simulink model "model4_linear"  (R2025b)
settings: Solver=ode23t  StartTime=0.0  StopTime=10  MaxStep=4e-5  RelTol=1e-3
undefined symbols (not defined in the file): current_con_ts, DiscIntNeverNeededParam, lin_current_con_Ki, lin_current_con_Kp, lin_dc_voltage_source, lin_gear_ratio, lin_lead, lin_motor_P_pole_pairs, lin_motor_P_rotorJ, lin_motor_P_statorLd, lin_motor_P_statorLq, lin_position_con_Kp, lin_velocity_con_Ki, lin_velocity_con_Kp, position_con_ts, velocity_con_ts
libraries: nesl_utility x11, fl_lib x9, ee_lib x7, mcbeeMathTransformLib x4, slpidlib x4, sdl_lib x1
settings Model: DataDictionary=model4_lin_data.sldd  Creator=HP-PC  LastModifiedBy=HP-PC
settings SolverCC: AutoInsertRateTranBlk=on  InsertRTBMode=Never (minimum delay)

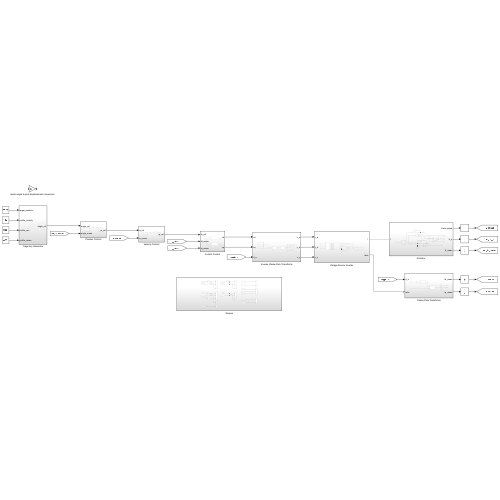
[thumbnail: Simulink's stored preview of the top-level diagram]
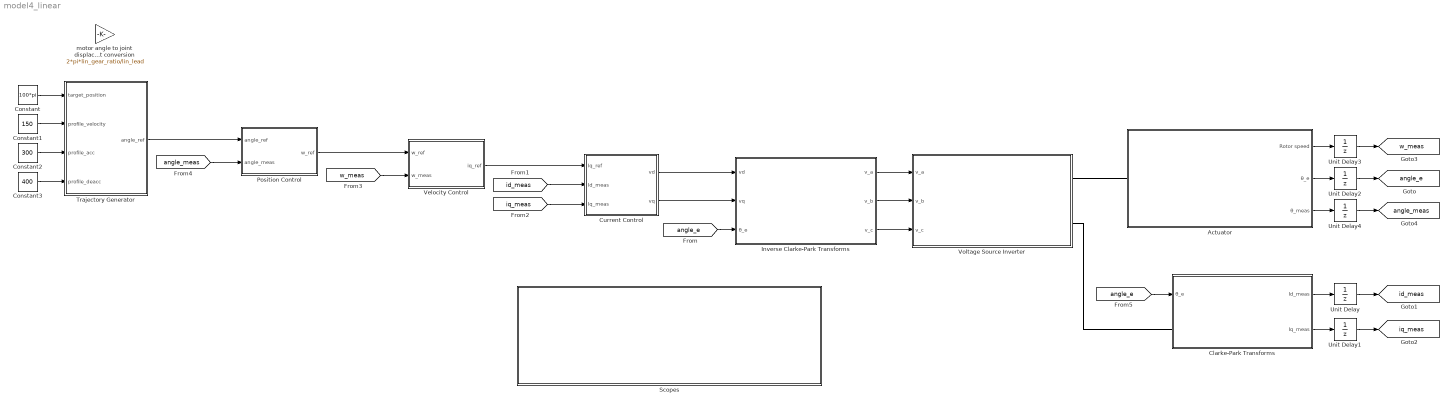
== system model4_linear ==
  Actuator : Subsystem
  Clarke-Park Transforms : Subsystem
  Constant : Constant  Value=100*pi
  Constant1 : Constant  Value=150
  Constant2 : Constant  Value=300
  Constant3 : Constant  Value=400
  Current Control : Subsystem
  Inverse Clarke-Park Transforms : Subsystem
  Position Control : Subsystem
  Scopes : Subsystem
  Trajectory Generator : Subsystem
  Unit Delay : UnitDelay  SampleTime=4e-5  HasFrameUpgradeWarning=on
  Unit Delay1 : UnitDelay  SampleTime=4e-5  HasFrameUpgradeWarning=on
  Unit Delay2 : UnitDelay  SampleTime=4e-5  HasFrameUpgradeWarning=on
  Unit Delay3 : UnitDelay  SampleTime=4e-4  HasFrameUpgradeWarning=on
  Unit Delay4 : UnitDelay  SampleTime=4e-4  HasFrameUpgradeWarning=on
  Velocity Control : Subsystem
  Voltage Source Inverter : Subsystem
  motor angle to joint displacement conversion : Gain  Gain=2*pi*lin_gear_ratio/lin_lead
  tag scope: angle_e=global, angle_meas=global, id_meas=global, iq_meas=global, w_meas=global
  wires:
  Inverse Clarke-Park Transforms/1(v_a) -> Voltage Source Inverter/1(v_a)
  Inverse Clarke-Park Transforms/2(v_b) -> Voltage Source Inverter/2(v_b)
  Inverse Clarke-Park Transforms/3(v_c) -> Voltage Source Inverter/3(v_c)
  Current Control/1(vd) -> Inverse Clarke-Park Transforms/1(vd)
  Current Control/2(vq) -> Inverse Clarke-Park Transforms/2(vq)
  Clarke-Park Transforms/1(Id_meas) -> Unit Delay/1
  Clarke-Park Transforms/2(Iq_meas) -> Unit Delay1/1
  Actuator/2(θ_e) -> Unit Delay2/1
  Unit Delay2/1 -> [angle_e]
  [angle_e] -> Inverse Clarke-Park Transforms/3(θ_e)
  Unit Delay/1 -> [id_meas]
  Unit Delay1/1 -> [iq_meas]
  [id_meas] -> Current Control/2(Id_meas)
  [iq_meas] -> Current Control/3(Iq_meas)
  Actuator/1(Rotor speed) -> Unit Delay3/1
  Unit Delay3/1 -> [w_meas]
  [w_meas] -> Velocity Control/2(w_meas)
  Position Control/1(w_ref) -> Velocity Control/1(w_ref)
  Actuator/3(θ_meas) -> Unit Delay4/1
  Unit Delay4/1 -> [angle_meas]
  [angle_meas] -> Position Control/2(angle_meas)
  Constant1/1 -> Trajectory Generator/2(profile_velocity)
  Constant2/1 -> Trajectory Generator/3(profile_acc)
  Constant3/1 -> Trajectory Generator/4(profile_deacc)
  Trajectory Generator/1(angle_ref) -> Position Control/1(angle_ref)
  Constant/1 -> Trajectory Generator/1(target_position)
  [angle_e] -> Clarke-Park Transforms/1(θ_e)
  Velocity Control/1(iq_ref) -> Current Control/1(Iq_ref)
  connections:
  Actuator/LConn1 -- Voltage Source Inverter/RConn1
  Voltage Source Inverter/RConn2 -- Clarke-Park Transforms/LConn1

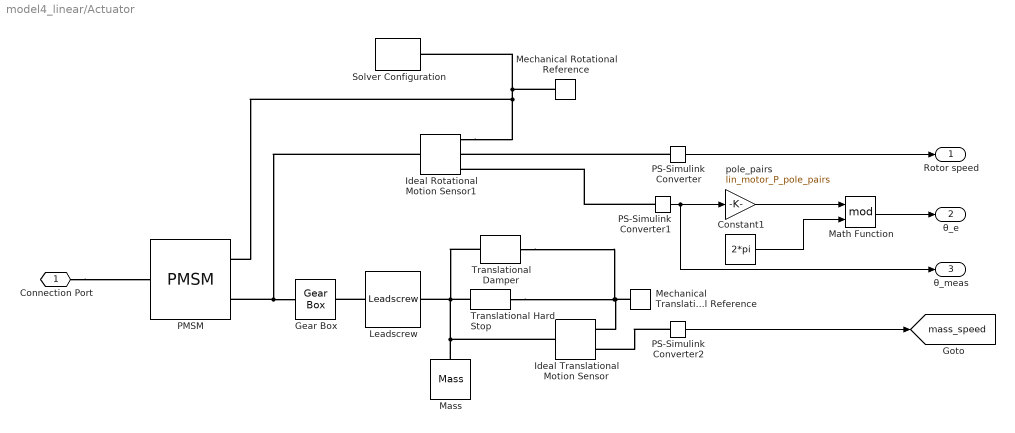
== system model4_linear/Actuator ==
  Constant1 : Constant  Value=2*pi
  Gear Box : fl_lib/Mechanical/Mechanisms/Gear Box  ratio=lin_gear_ratio  t_in_specify=off  t_in_priority=None  t_in=0 N*m  t_in_nominal_specify=off  t_in_nominal_value=1  t_in_nominal_unit=N*m  t_out_specify=off  t_out_priority=None  t_out=0 N*m  t_out_nominal_specify=off  t_out_nominal_value=1  t_out_nominal_unit=N*m
  Ideal Rotational Motion Sensor1 : fl_lib/Mechanical/Mechanical Sensors/Ideal Rotational Motion Sensor  reference=foundation.enum.MeasurementReference.difference  acceleration_port=false  velocity_port=true  position_port=true  wrap_angle=false  offset=0 rad
  Ideal Translational Motion Sensor : fl_lib/Mechanical/Mechanical Sensors/Ideal Translational Motion Sensor  reference=foundation.enum.MeasurementReference.difference  acceleration_port=false  velocity_port=true  position_port=false  offset=0 m
      settings: InternalSimscapePortConfiguration="{\"Bottom\":[],\"Left\":[{\"id\":\"R\",\"label\":\"R\",\"type\":\"foundation.mechanical.translational.translational\"}],\"Right\":[{\"id\":\"C\",\"label\":\"C\",\"type\":\"foundation.mechanical.translational.translational\"},{\"id\":\"V\",\"label\":\"V\",\"type\":\"output\"}],\"Top\":[]}"
  Leadscrew : sdl_lib/Gears/Rotational- Translational/Leadscrew  Lead=lin_lead m  helix_type=sdl.enum.handedness.right  friction_model=sdl.enum.gear_friction.constant  friction_parameterization=sdl.enum.frictionParameterization.efficiencies  lambda=15 deg  alpha=14.5 deg  fr_coeff=0.08  eff_sn=lin_screwnut_efficiency  eff_ns=lin_screwnut_efficiency  temperature_TLU=[280, 300, 320] K  efficiency_sn_TLU=[.75, .65, .6]  efficiency_ns_TLU=[.5, .45, .4]  pwr_thr=0.001 W  mu_visc=0 N*m*s/rad  thermal_mass=50 J/K  temperature_specify=off  temperature_priority=High  temperature=300 K  temperature_nominal_specify=off  temperature_nominal_value=1  temperature_nominal_unit=K
      settings: InternalSimscapePortConfiguration="{\"Bottom\":[],\"Left\":[{\"id\":\"S\",\"label\":\"S\",\"type\":\"foundation.mechanical.rotational.rotational\"}],\"Right\":[{\"id\":\"N\",\"label\":\"N\",\"type\":\"foundation.mechanical.translational.translational\"}],\"Top\":[]}"
  Mass : fl_lib/Mechanical/Translational Elements/Mass  mass=1 kg  num_ports=foundation.enum.numPorts2.one  v_specify=off  v_priority=High  v=0 m/s  v_nominal_specify=off  v_nominal_value=1  v_nominal_unit=m/s  f_specify=off  f_priority=None  f=0 N  f_nominal_specify=off  f_nominal_value=1  f_nominal_unit=N
  Math Function : Math  Operator=mod
  Mechanical Rotational Reference : fl_lib/Mechanical/Rotational Elements/Mechanical Rotational Reference
  Mechanical Translational Reference : fl_lib/Mechanical/Translational Elements/Mechanical Translational Reference
  PMSM : ee_lib/Electromechanical/Permanent Magnet/PMSM  port_option=ee.enum.threePhasePort.composite  winding_type=ee.enum.electromech.statorconfiguration.wye  machine_param=ee.enum.pmsm.parameterization.constant  nPolePairs=lin_motor_P_pole_pairs  pmflux_param=ee.enum.pmflux.torqueconstant  pm_flux_linkage=0.03 Wb  torque_constant=lin_motor_P_torqueK N*m/A  back_emf_constant=0.18 V*s/rad  stator_param=ee.enum.statorparam.LdLqL0  Ld=lin_motor_P_statorLd H  Lq=lin_motor_P_statorLq H  idVec=[-200, 0, 200] A  iqVec=[-200, 0, 200] A  LdMatrix=0.0002 * ones(3, 3) H  LqMatrix=0.0002 * ones(3, 3) H  PmMatrix=0.1 * ones(3, 3) Wb  ktMatrix=0.18 * ones(3, 3) N*m/A  keMatrix=0.18 * ones(3, 3) V*s/rad  L0=0.00016 H  Ls=0.0002 H  Lm=-0.00002 H  Ms=0.00002 H  Rs=lin_motor_P_statorR Ohm  zero_sequence=ee.enum.park.zerosequence.exclude  axes_param=ee.enum.rotorangle.daxis  loss_param=ee.enum.ironloss.none  losses_oc=[0, 0, 0] W  losses_sc=[0, 0, 0] W  f_losses=60 Hz  Isc_losses=95 A  J=lin_motor_P_rotorJ kg*m^2  lam=0 N*m*s/rad  i_d_specify=off  i_d_priority=None  i_d=0 A  i_d_nominal_specify=off  i_d_nominal_value=1  i_d_nominal_unit=A  i_q_specify=off  i_q_priority=None  i_q=0 A  i_q_nominal_specify=off  i_q_nominal_value=1  i_q_nominal_unit=A  torque_specify=off  torque_priority=None  torque=0 N*m  torque_nominal_specify=off  torque_nominal_value=1  torque_nominal_unit=N*m  angular_velocity_specify=off  angular_velocity_priority=High  angular_velocity=0 rpm  angular_velocity_nominal_specify=off  angular_velocity_nominal_value=1  angular_velocity_nominal_unit=rpm  angular_position_specify=off  angular_position_priority=High  angular_position=0 deg  angular_position_nominal_specify=off  angular_position_nominal_value=1  angular_position_nominal_unit=deg  alpha=3.93e-3 1/K  alpha_flux=-0.001 1/K  Tmeas=298.15 K  stator_thermal_mass=100 J/K  rotor_thermal_mass=200 J/K  Rm_percent_rotor=90  Rd_percent_rotor=30  temperatureA_specify=off  temperatureA_priority=High  temperatureA=25 degC  temperatureA_nominal_specify=off  temperatureA_nominal_value=1  temperatureA_nominal_unit=degC  temperatureB_specify=off  temperatureB_priority=High  temperatureB=25 degC  temperatureB_nominal_specify=off  temperatureB_nominal_value=1  temperatureB_nominal_unit=degC  temperatureC_specify=off  temperatureC_priority=High  temperatureC=25 degC  temperatureC_nominal_specify=off  temperatureC_nominal_value=1  temperatureC_nominal_unit=degC  temperatureR_specify=off  temperatureR_priority=High  temperatureR=25 degC  temperatureR_nominal_specify=off  temperatureR_nominal_value=1  temperatureR_nominal_unit=degC
      settings: InternalSimscapePortConfiguration="{\"Bottom\":[],\"Left\":[{\"id\":\"N\",\"label\":\"~\",\"type\":\"foundation.electrical.three_phase\"}],\"Right\":[{\"id\":\"R\",\"label\":\"R\",\"type\":\"foundation.mechanical.rotational.rotational\"},{\"id\":\"C\",\"label\":\"C\",\"type\":\"foundation.mechanical.rotational.rotational\"}],\"Top\":[]}"
  PS-Simulink Converter : nesl_utility/PS-Simulink Converter  PhysicalDomain=network_engine_domain  SubClassName=ps_output  LeftPortType=input  RightPortType=output  PseudoPeriodic=off  Frequencies=[]  VectorFormat=inherit  Unit=rad/s  AffineConversion=off
  PS-Simulink Converter1 : nesl_utility/PS-Simulink Converter  PhysicalDomain=network_engine_domain  SubClassName=ps_output  LeftPortType=input  RightPortType=output  PseudoPeriodic=off  Frequencies=[]  VectorFormat=inherit  Unit=rad  AffineConversion=off
  PS-Simulink Converter2 : nesl_utility/PS-Simulink Converter  PhysicalDomain=network_engine_domain  SubClassName=ps_output  LeftPortType=input  RightPortType=output  PseudoPeriodic=off  Frequencies=[]  VectorFormat=inherit  Unit=inherit  AffineConversion=off
  Solver Configuration : nesl_utility/Solver Configuration  PhysicalDomain=network_engine_domain  SubClassName=solver  LeftPortType=input  RightPortType=generic  Tones=[]  Harmonics=[]  SimulateNoise=off  Profile=off  UseLocalSampling=off  EnableSwitchedLinearOptims=on  FrequencyDomain=off  UseCCode=off  RelTol=0.001  AbsTol=0.001  MinStep=1e-09  ToWorkspace=off  RevertToSquareIcSolve=off  NumHomotopyIterations=100  PhasorMode=off  PhasorModeNumHarmonics=1  ConsistencySolver=NEWTON_XTOL_AFTER_FTOL  IndexReductionMethod=DerivativeReplacement  DoDC=off  ResidualTolerance=1e-09  ConsistencyTolSource=GLOBAL  ConsistencyAbsTol=0.001  ConsistencyRelTol=0.001  ConsistencyTolFactor=0.001  UseLocalSolver=off  LocalSolverChoice=NE_BACKWARD_EULER_ADVANCER  ResolveIndetEquations=on  FunctionEvalNumThread=1  LocalSolverSampleTime=0.001  DoFixedCost=off  MaxNonlinIter=3  MaxModeIter=2  ComputeImpulses=off  ImpulseIterations=2  LinearAlgebra=auto  LinearAlgebraNumThread=0  EquationFormulation=NE_TIME_EF  DelaysMemoryBudget=1024  AutomaticFiltering=on  FilteringTimeConstant=0.001  PartitionStorageMethod=AS_NEEDED  PartitionMemoryBudget=1024  PartitionMethod=ROBUST  MultibodyUseLocalSolver=off  MultibodyLocalSolverChoice=ODE1  MultibodyLocalSolverSampleTime=0.001
  Translational Damper : fl_lib/Mechanical/Translational Elements/Translational Damper  D=10 N*s/m  v_specify=off  v_priority=None  v=0 m/s  v_nominal_specify=off  v_nominal_value=1  v_nominal_unit=m/s  f_specify=off  f_priority=None  f=0 N  f_nominal_specify=off  f_nominal_value=1  f_nominal_unit=N
  Translational Hard Stop : fl_lib/Mechanical/Translational Elements/Translational Hard Stop  upper_bnd=0.05 m  lower_bnd=-0.05 m  model=simscape.enum.hardstop.smooth  stiff_up=1e6 N/m  stiff_low=1e6 N/m  D_up=150 N*s/m  D_low=150 N*s/m  transition=0.1 mm  coeff_rest=0.7  v_tol=0.001 m/s  f_tol=0.001 N  v_specify=off  v_priority=None  v=0 m/s  v_nominal_specify=off  v_nominal_value=1  v_nominal_unit=m/s  f_specify=off  f_priority=None  f=0 N  f_nominal_specify=off  f_nominal_value=1  f_nominal_unit=N  x_specify=off  x_priority=High  x=0 m  x_nominal_specify=off  x_nominal_value=1  x_nominal_unit=m  M_specify=off  M_priority=None  M=0
  pole_pairs : Gain  Gain=lin_motor_P_pole_pairs
  Connection Port : PMIOPort  Side=Left
  Rotor speed : Outport
  θ_e : Outport  Port=2
  θ_meas : Outport  Port=3
  tag scope: mass_speed=global
  wires:
  PS-Simulink Converter/1 -> Rotor speed/1
  pole_pairs/1 -> Math Function/1
  Constant1/1 -> Math Function/2
  PS-Simulink Converter1/1 -> θ_meas/1, pole_pairs/1
  Math Function/1 -> θ_e/1
  PS-Simulink Converter2/1 -> [mass_speed]
  connections:
  Mechanical Rotational Reference/LConn1 -- Ideal Rotational Motion Sensor1/RConn1 -- PMSM/RConn2 -- Solver Configuration/RConn1
  PS-Simulink Converter/LConn1 -- Ideal Rotational Motion Sensor1/RConn2
  Connection Port/RConn1 -- PMSM/LConn1
  Ideal Rotational Motion Sensor1/LConn1 -- Gear Box/LConn1 -- PMSM/RConn1
  PS-Simulink Converter1/LConn1 -- Ideal Rotational Motion Sensor1/RConn3
  Leadscrew/LConn1 -- Gear Box/RConn1
  Translational Damper/LConn1 -- Ideal Translational Motion Sensor/LConn1 -- Mass/LConn1 -- Leadscrew/RConn1 -- Translational Hard Stop/LConn1
  Mechanical Translational Reference/LConn1 -- Translational Hard Stop/RConn1 -- Translational Damper/RConn1 -- Ideal Translational Motion Sensor/RConn1
  PS-Simulink Converter2/LConn1 -- Ideal Translational Motion Sensor/RConn2

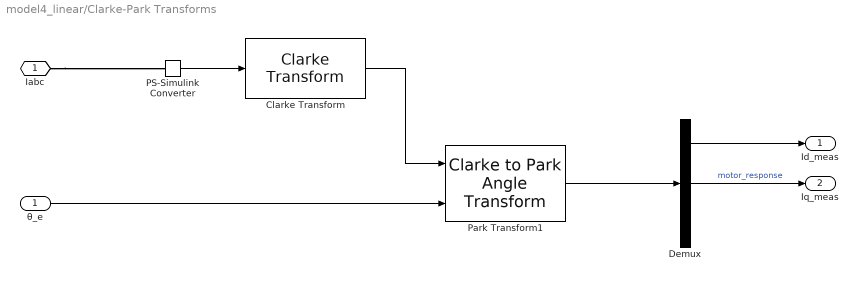
== system model4_linear/Clarke-Park Transforms ==
  θ_e : Inport
  Clarke Transform : mcbeeMathTransformLib/Clarke Transform  VariantControl=Variant2  PowerInvariant=off  UseWithEmbedded=on  PhaseInput=Three inputs
      settings: LibrarySourceBlock=mcblib/Controls/Math Transforms/Clarke Transform
  Demux : Demux  Outputs=3
  PS-Simulink Converter : nesl_utility/PS-Simulink Converter  PhysicalDomain=network_engine_domain  SubClassName=ps_output  LeftPortType=input  RightPortType=output  PseudoPeriodic=off  Frequencies=[]  VectorFormat=inherit  Unit=inherit  AffineConversion=off
  Park Transform1 : mcbeeMathTransformLib/Clarke to Park Angle Transform  AxisAlignment=D-axis  UseWithEmbedded=on  PhaseInput=Three inputs  ThetaInput=Electrical position  AngleInput=Radians  N_points=1024
      settings: LibrarySourceBlock=mcblib/Controls/Math Transforms/Park Transform
  Iabc : PMIOPort  Side=Left
  Id_meas : Outport
  Iq_meas : Outport  Port=2
  wires:
  PS-Simulink Converter/1 -> Clarke Transform/1
  Clarke Transform/1 -> Park Transform1/1
  Park Transform1/1 -> Demux/1
  Demux/1 -> Id_meas/1
  Demux/2 -> Iq_meas/1  "motor_response"
  θ_e/1 -> Park Transform1/2
  connections:
  Iabc/RConn1 -- PS-Simulink Converter/LConn1

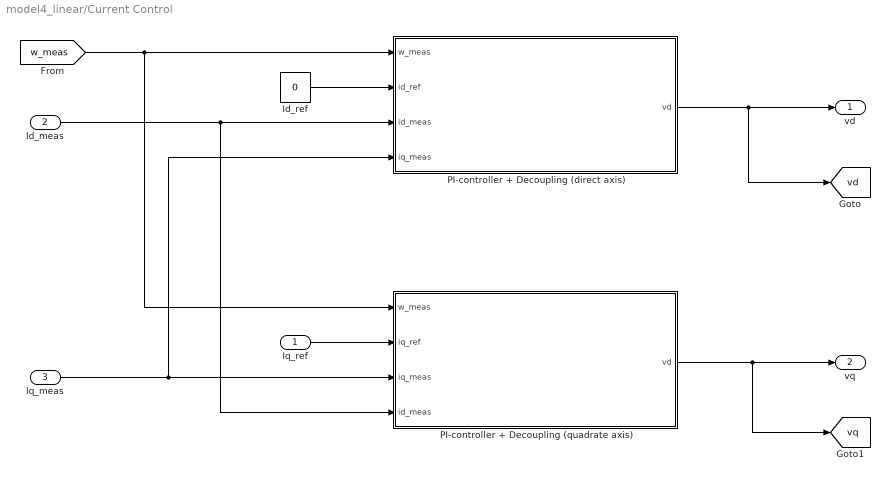
== system model4_linear/Current Control ==
  Iq_ref : Inport
  Id_meas : Inport  Port=2
  Iq_meas : Inport  Port=3
  Id_ref : Constant  Value=0
  PI-controller + Decoupling (direct axis) : Subsystem
  PI-controller + Decoupling (quadrate axis) : Subsystem
  vd : Outport
  vq : Outport  Port=2
  tag scope: vd=global, vq=global
  wires:
  [w_meas] -> PI-controller + Decoupling (quadrate axis)/1(w_meas), PI-controller + Decoupling (direct axis)/1(w_meas)
  Id_ref/1 -> PI-controller + Decoupling (direct axis)/2(id_ref)
  Id_meas/1 -> PI-controller + Decoupling (quadrate axis)/4(id_meas), PI-controller + Decoupling (direct axis)/3(id_meas)
  PI-controller + Decoupling (quadrate axis)/1(vd) -> [vq], vq/1
  PI-controller + Decoupling (direct axis)/1(vd) -> [vd], vd/1
  Iq_ref/1 -> PI-controller + Decoupling (quadrate axis)/2(iq_ref)
  Iq_meas/1 -> PI-controller + Decoupling (direct axis)/4(iq_meas), PI-controller + Decoupling (quadrate axis)/3(iq_meas)

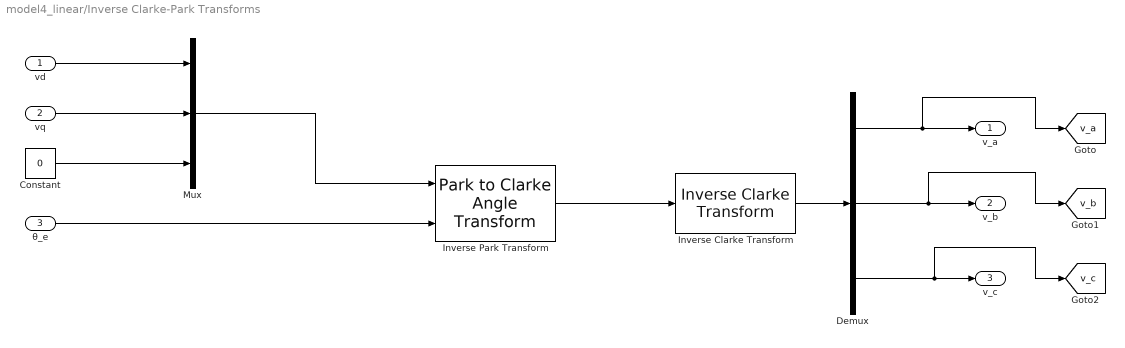
== system model4_linear/Inverse Clarke-Park Transforms ==
  vd : Inport
  vq : Inport  Port=2
  θ_e : Inport  Port=3
  Constant : Constant  Value=0
  Demux : Demux  Outputs=3
  Inverse Clarke Transform : mcbeeMathTransformLib/Inverse Clarke Transform  PowerInvariant=off  UseWithEmbedded=on  PhaseInput=Three inputs
      settings: LibrarySourceBlock=mcblib/Controls/Math Transforms/Inverse Clarke Transform
  Inverse Park Transform : mcbeeMathTransformLib/Park to Clarke Angle Transform  AxisAlignment=D-axis  UseWithEmbedded=on  PhaseInput=Three inputs  ThetaInput=Electrical position  AngleInput=Radians  N_points=1024
      settings: LibrarySourceBlock=mcblib/Controls/Math Transforms/Inverse Park Transform
  Mux : Mux  Inputs=3
  v_a : Outport
  v_b : Outport  Port=2
  v_c : Outport  Port=3
  tag scope: v_a=global, v_b=global, v_c=global
  wires:
  Inverse Park Transform/1 -> Inverse Clarke Transform/1
  θ_e/1 -> Inverse Park Transform/2
  vd/1 -> Mux/1
  vq/1 -> Mux/2
  Constant/1 -> Mux/3
  Demux/3 -> [v_c], v_c/1
  Demux/2 -> [v_b], v_b/1
  Demux/1 -> [v_a], v_a/1
  Inverse Clarke Transform/1 -> Demux/1
  Mux/1 -> Inverse Park Transform/1

== system model4_linear/Position Control ==
  angle_ref : Inport
  angle_meas : Inport  Port=2
  PID Controller : slpidlib/PID Controller  Controller=P  Form=Parallel  TimeDomain=Discrete-time  UseExternalTs=off  SampleTime=position_con_ts  IntegratorMethod=Forward Euler  FilterMethod=Forward Euler  ControllerParametersSource=internal  P=lin_position_con_Kp  I=1  UseKiTs=off  D=0  UseExternalDerivativeSource=off  N=100  UseFilter=on  TunerSelectOption=Transfer Function Based (PID Tuner App)  InitialConditionSource=internal  InitialConditionForIntegrator=0  InitialConditionForFilter=0  DifferentiatorICPrevScaledInput=0  ExternalReset=none  TrackingMode=off  Kt=1  LimitOutput=on  SatLimitsSource=internal  UpperSaturationLimit=837  LowerSaturationLimit=-837  LinearizeAsGain=on  AntiWindupMode=none  Kb=1  LimitIntegrator=off  UpperIntegratorSaturationLimit=inf  LowerIntegratorSaturationLimit=-inf  POutMin=[]  POutMax=[]  IOutMin=[]  IOutMax=[]  DOutMin=[]  DOutMax=[]  NOutMin=[]  NOutMax=[]  SumOutMin=[]  SumOutMax=[]  SaturationOutMin=[]  SaturationOutMax=[]  PParamMin=[]  PParamMax=[]  IParamMin=[]  IParamMax=[]  DParamMin=[]  DParamMax=[]  NParamMin=[]  NParamMax=[]  KbParamMin=[]  KbParamMax=[]  KtParamMin=[]  KtParamMax=[]  KbOutMin=[]  KbOutMax=[]  KtOutMin=[]  KtOutMax=[]  IntegratorOutMin=[]  IntegratorOutMax=[]  FilterOutMin=[]  FilterOutMax=[]  SumI1OutMin=[]  SumI1OutMax=[]  SumI2OutMin=[]  SumI2OutMax=[]  SumI3OutMin=[]  SumI3OutMax=[]  SumI4OutMin=[]  SumI4OutMax=[]  SumDOutMin=[]  SumDOutMax=[]  DifferentiatorOutMin=[]  DifferentiatorOutMax=[]  FilterDiffOutCoefMin=[]  FilterDiffOutCoefMax=[]  ReciprocalOutMin=[]  ReciprocalOutMax=[]  SumDenOutMin=[]  SumDenOutMax=[]  SumNumOutMin=[]  SumNumOutMax=[]  DivideOutMin=[]  DivideOutMax=[]  UdiffTsProdOutMin=[]  UdiffTsProdOutMax=[]  NTsProdOutMin=[]  NTsProdOutMax=[]  UintegralTsProdOutMin=[]  UintegralTsProdOutMax=[]  UngainTsProdOutMin=[]  UngainTsProdOutMax=[]  ClampingZeroOutDataTypeStr=Inherit: Inherit via back propagation  ClampingZeroOutMin=[]  ClampingZeroOutMax=[]  FilterDenConstantOutDataTypeStr=Inherit: Inherit via back propagation  FilterDenConstantOutMin=[]  FilterDenConstantOutMax=[]  PCopyOutDataTypeStr=Inherit: Inherit via back propagation  PCopyOutMin=[]  PCopyOutMax=[]  NCopyOutDataTypeStr=Inherit: Inherit via back propagation  NCopyOutMin=[]  NCopyOutMax=[]  IntegratorContinuousStateAttributes=''  IntegratorStateMustResolveToSignalObject=off  IntegratorRTWStateStorageClass=Auto  FilterContinuousStateAttributes=''  FilterStateMustResolveToSignalObject=off  FilterRTWStateStorageClass=Auto  ParallelPVariant=InternalParameters  IdealPVariant=Disabled  IVariant=Disabled  DVariant=Disabled  IntegratorVariant=Disabled  SatVariant=Enabled  AWVariant=Disabled  PCopyVariant=Disabled  TRVariant=Disabled  FdbkBlocksVariant=Forward  IdealPFdbkVariant=Disabled  SatFdbkVariant=Disabled  DerivativeFilterVariant=Disabled  NVariant=Disabled  NCopyVariant=Disabled_SignalSpec  FilterICVariant=Disabled  IntegratorICVariant=Disabled  ExternalResetVariant=Disabled  TRSumVariant=Passthrough  SumFdbkVariant=Disabled  SumVariant=Passthrough_P  TsampFilterVariant=InternalTs  TsampNgainVariant=Passthrough  TsampIntegralVariant=Disabled_SignalSpec  ExternalSaturationOutDataTypeStr=Inherit: Same as second input  DerivativeSourceVariant=Disabled  PreIntVariant=InternalPreInt
  Sum : Sum  Inputs=|+-
  w_ref : Outport
  tag scope: w_ref=global
  wires:
  angle_ref/1 -> Sum/1
  angle_meas/1 -> Sum/2
  Sum/1 -> PID Controller/1
  PID Controller/1 -> [w_ref], w_ref/1

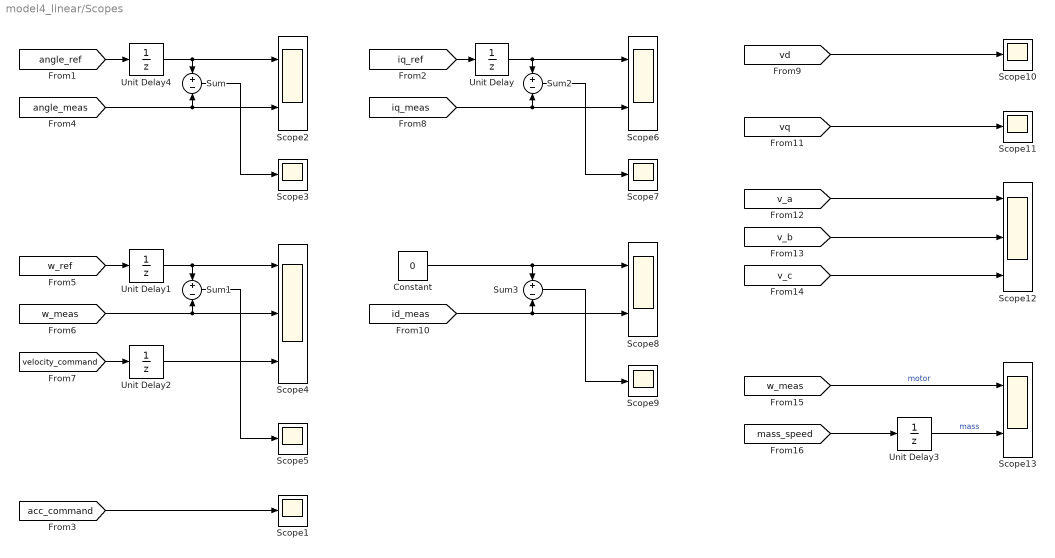
== system model4_linear/Scopes ==
  Constant : Constant  Value=0
  Scope{1,3,5,7,9..11} (7 alike) : Scope
      Scope1 settings: ActiveDisplayYMinimum=-37.499999999999993  ActiveDisplayYMaximum=337.5  DataLoggingVariableName=ScopeData7
      Scope10 settings: ActiveDisplayYMinimum=-0.0423730264107981  ActiveDisplayYMaximum=0.0047081140456442325  DataLoggingVariableName=ScopeData2
      Scope11 settings: ActiveDisplayYMinimum=-2.2499999999999996  ActiveDisplayYMaximum=20.25  DataLoggingVariableName=ScopeData12
      Scope3 settings: ActiveDisplayYMinimum=-1.8674948083140914  ActiveDisplayYMaximum=16.807453274826827  DataLoggingVariableName=ScopeData9
      Scope5 settings: ActiveDisplayYMinimum=-43.62771491917448  ActiveDisplayYMaximum=43.84143571921804  DataLoggingVariableName=ScopeData10
      Scope7 settings: ActiveDisplayYMinimum=-0.25302414136209772  ActiveDisplayYMaximum=2.2503360157007775  DataLoggingVariableName=ScopeData6
      Scope9 settings: ActiveDisplayYMinimum=-2.4518695185843924E-5  ActiveDisplayYMaximum=2.724299465616759E-6  DataLoggingVariableName=ScopeData11
  Scope12 : Scope  NumInputPorts=3
      settings: ActiveDisplayYMinimum=-22.826049332319911  ActiveDisplayYMaximum=22.826210037477324  DataLoggingVariableName=ScopeData13
  Scope{2,6,8,13} (4 alike) : Scope  NumInputPorts=2
      Scope13 settings: ActiveDisplayYMinimum=381.91543442216278  ActiveDisplayYMaximum=436.89236308010203
      Scope2 settings: ActiveDisplayYMinimum=-149.83096756253232  ActiveDisplayYMaximum=430.36800139661909  DataLoggingVariableName=ScopeData8
      Scope6 settings: ActiveDisplayYMinimum=-3.8794713807528716  ActiveDisplayYMaximum=4.0910523756392081  DataLoggingVariableName=ScopeData5
      Scope8 settings: ActiveDisplayYMinimum=-0.026373140535182117  ActiveDisplayYMaximum=0.072491403258309661  DataLoggingVariableName=ScopeData3
  Scope4 : Scope  NumInputPorts=3
      settings: ActiveDisplayYMinimum=-12.813947189558023  ActiveDisplayYMaximum=115.32552470602224  DataLoggingVariableName=ScopeData4
  Sum{,1..3} (4 alike) : Sum  Inputs=+-
  Unit Delay : UnitDelay  SampleTime=4e-5  HasFrameUpgradeWarning=on
  Unit Delay{1..4} (4 alike) : UnitDelay  SampleTime=4e-4  HasFrameUpgradeWarning=on
  wires:
  [acc_command] -> Scope1/1
  [angle_meas] -> Scope2/2, Sum/2
  [angle_ref] -> Unit Delay4/1
  Sum/1 -> Scope3/1
  [w_ref] -> Unit Delay1/1
  Sum1/1 -> Scope5/1
  [w_meas] -> Scope4/2, Sum1/2
  [velocity_command] -> Unit Delay2/1
  [iq_ref] -> Unit Delay/1
  Sum2/1 -> Scope7/1
  [iq_meas] -> Scope6/2, Sum2/2
  Constant/1 -> Scope8/1, Sum3/1
  Sum3/1 -> Scope9/1
  [id_meas] -> Scope8/2, Sum3/2
  [vd] -> Scope10/1
  [vq] -> Scope11/1
  [v_a] -> Scope12/1
  [v_b] -> Scope12/2
  [v_c] -> Scope12/3
  [w_meas] -> Scope13/1  "motor"
  [mass_speed] -> Unit Delay3/1
  Unit Delay4/1 -> Scope2/1, Sum/1
  Unit Delay1/1 -> Scope4/1, Sum1/1
  Unit Delay2/1 -> Scope4/3
  Unit Delay3/1 -> Scope13/2  "mass"
  Unit Delay/1 -> Scope6/1, Sum2/1

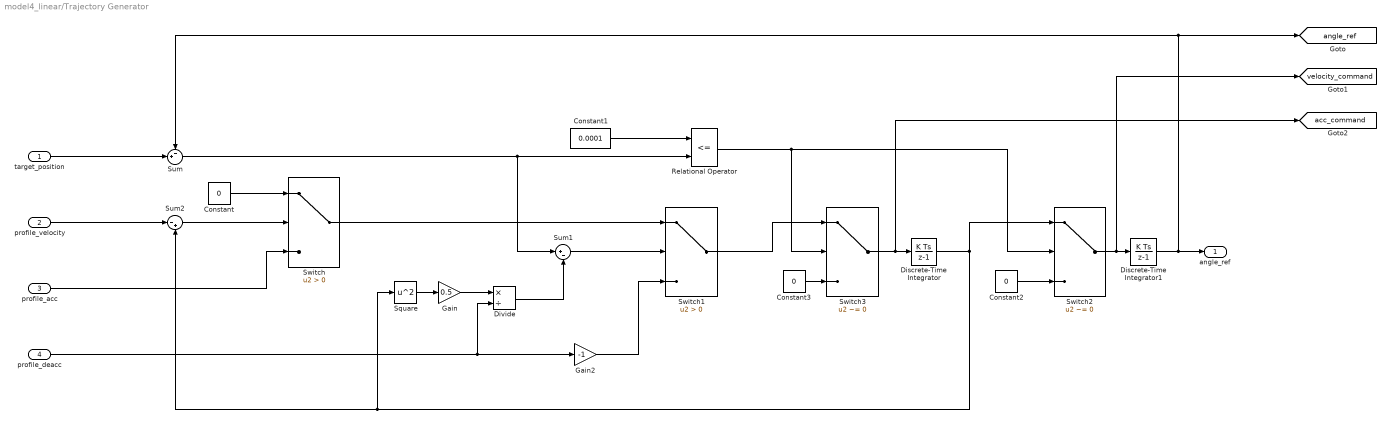
== system model4_linear/Trajectory Generator ==
  target_position : Inport
  profile_velocity : Inport  Port=2
  profile_acc : Inport  Port=3
  profile_deacc : Inport  Port=4
  Constant : Constant  Value=0
  Constant1 : Constant  Value=0.0001
  Constant2 : Constant  Value=0
  Constant3 : Constant  Value=0
  Discrete-Time Integrator : DiscreteIntegrator  SampleTime=4e-4  ICPrevOutput=DiscIntNeverNeededParam  ICPrevScaledInput=DiscIntNeverNeededParam
  Discrete-Time Integrator1 : DiscreteIntegrator  SampleTime=4e-4  ICPrevOutput=DiscIntNeverNeededParam  ICPrevScaledInput=DiscIntNeverNeededParam
  Divide : Product  Inputs=*/
  Gain : Gain  Gain=0.5
  Gain2 : Gain  Gain=-1
  Relational Operator : RelationalOperator  Operator=<=  OutDataTypeStr=boolean  RndMeth=Simplest  InputSameDT=off
  Square : Math  Operator=square
  Sum : Sum  Inputs=-+|
  Sum1 : Sum  Inputs=|+-
  Sum2 : Sum  Inputs=|-+
  Switch : Switch  Criteria=u2 > Threshold  SaturateOnIntegerOverflow=off  InputSameDT=off
  Switch1 : Switch  Criteria=u2 > Threshold  SaturateOnIntegerOverflow=off  InputSameDT=off
  Switch2 : Switch  Criteria=u2 ~= 0  SaturateOnIntegerOverflow=off  InputSameDT=off
  Switch3 : Switch  Criteria=u2 ~= 0  SaturateOnIntegerOverflow=off  InputSameDT=off
  angle_ref : Outport
  tag scope: acc_command=global, angle_ref=global, velocity_command=global
  wires:
  Square/1 -> Gain/1
  Gain/1 -> Divide/1
  Sum1/1 -> Switch1/2
  Divide/1 -> Sum1/2
  Sum/1 -> Sum1/1, Relational Operator/2
  Sum2/1 -> Switch/2
  profile_velocity/1 -> Sum2/1
  profile_acc/1 -> Switch/3
  Constant/1 -> Switch/1
  Switch/1 -> Switch1/1
  Discrete-Time Integrator/1 -> Switch2/1, Sum2/2, Square/1
  Discrete-Time Integrator1/1 -> [angle_ref], Sum/1, angle_ref/1
  profile_deacc/1 -> Divide/2, Gain2/1
  Constant1/1 -> Relational Operator/1
  target_position/1 -> Sum/2
  Switch2/1 -> [velocity_command], Discrete-Time Integrator1/1
  Relational Operator/1 -> Switch3/2, Switch2/2
  Constant2/1 -> Switch2/3
  Gain2/1 -> Switch1/3
  Constant3/1 -> Switch3/3
  Switch3/1 -> [acc_command], Discrete-Time Integrator/1
  Switch1/1 -> Switch3/1

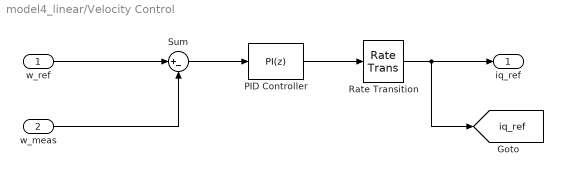
== system model4_linear/Velocity Control ==
  w_ref : Inport
  w_meas : Inport  Port=2
  PID Controller : slpidlib/PID Controller  Controller=PI  Form=Parallel  TimeDomain=Discrete-time  UseExternalTs=off  SampleTime=velocity_con_ts  IntegratorMethod=Forward Euler  FilterMethod=Forward Euler  ControllerParametersSource=internal  P=lin_velocity_con_Kp  I=lin_velocity_con_Ki  UseKiTs=off  D=0  UseExternalDerivativeSource=off  N=100  UseFilter=on  TunerSelectOption=Transfer Function Based (PID Tuner App)  InitialConditionSource=internal  InitialConditionForIntegrator=0  InitialConditionForFilter=0  DifferentiatorICPrevScaledInput=0  ExternalReset=none  TrackingMode=off  Kt=1  LimitOutput=on  SatLimitsSource=internal  UpperSaturationLimit=+3.36  LowerSaturationLimit=-3.36  LinearizeAsGain=on  AntiWindupMode=clamping  Kb=1  LimitIntegrator=off  UpperIntegratorSaturationLimit=inf  LowerIntegratorSaturationLimit=-inf  POutMin=[]  POutMax=[]  IOutMin=[]  IOutMax=[]  DOutMin=[]  DOutMax=[]  NOutMin=[]  NOutMax=[]  SumOutMin=[]  SumOutMax=[]  SaturationOutMin=[]  SaturationOutMax=[]  PParamMin=[]  PParamMax=[]  IParamMin=[]  IParamMax=[]  DParamMin=[]  DParamMax=[]  NParamMin=[]  NParamMax=[]  KbParamMin=[]  KbParamMax=[]  KtParamMin=[]  KtParamMax=[]  KbOutMin=[]  KbOutMax=[]  KtOutMin=[]  KtOutMax=[]  IntegratorOutMin=[]  IntegratorOutMax=[]  FilterOutMin=[]  FilterOutMax=[]  SumI1OutMin=[]  SumI1OutMax=[]  SumI2OutMin=[]  SumI2OutMax=[]  SumI3OutMin=[]  SumI3OutMax=[]  SumI4OutMin=[]  SumI4OutMax=[]  SumDOutMin=[]  SumDOutMax=[]  DifferentiatorOutMin=[]  DifferentiatorOutMax=[]  FilterDiffOutCoefMin=[]  FilterDiffOutCoefMax=[]  ReciprocalOutMin=[]  ReciprocalOutMax=[]  SumDenOutMin=[]  SumDenOutMax=[]  SumNumOutMin=[]  SumNumOutMax=[]  DivideOutMin=[]  DivideOutMax=[]  UdiffTsProdOutMin=[]  UdiffTsProdOutMax=[]  NTsProdOutMin=[]  NTsProdOutMax=[]  UintegralTsProdOutMin=[]  UintegralTsProdOutMax=[]  UngainTsProdOutMin=[]  UngainTsProdOutMax=[]  ClampingZeroOutDataTypeStr=Inherit: Inherit via back propagation  ClampingZeroOutMin=[]  ClampingZeroOutMax=[]  FilterDenConstantOutDataTypeStr=Inherit: Inherit via back propagation  FilterDenConstantOutMin=[]  FilterDenConstantOutMax=[]  PCopyOutDataTypeStr=Inherit: Inherit via back propagation  PCopyOutMin=[]  PCopyOutMax=[]  NCopyOutDataTypeStr=Inherit: Inherit via back propagation  NCopyOutMin=[]  NCopyOutMax=[]  IntegratorContinuousStateAttributes=''  IntegratorStateMustResolveToSignalObject=off  IntegratorRTWStateStorageClass=Auto  FilterContinuousStateAttributes=''  FilterStateMustResolveToSignalObject=off  FilterRTWStateStorageClass=Auto  ParallelPVariant=InternalParameters  IdealPVariant=Disabled  IVariant=InternalParameters  DVariant=Disabled  IntegratorVariant=Discrete  SatVariant=Enabled  AWVariant=DiscClampingParallel  PCopyVariant=Disabled  TRVariant=Disabled  FdbkBlocksVariant=Forward  IdealPFdbkVariant=Disabled  SatFdbkVariant=Disabled  DerivativeFilterVariant=Disabled  NVariant=Disabled  NCopyVariant=Disabled_SignalSpec  FilterICVariant=Disabled  IntegratorICVariant=InternalICs  ExternalResetVariant=Disabled  TRSumVariant=Passthrough  SumFdbkVariant=Disabled  SumVariant=Sum_PI  TsampFilterVariant=InternalTs  TsampNgainVariant=Passthrough  TsampIntegralVariant=Disabled_SignalSpec  ExternalSaturationOutDataTypeStr=Inherit: Same as second input  DerivativeSourceVariant=Disabled  PreIntVariant=InternalPreInt
  Rate Transition : RateTransition  Deterministic=off  OutPortSampleTime=4e-5
  Sum : Sum  Inputs=|+-
  iq_ref : Outport
  tag scope: iq_ref=global
  wires:
  PID Controller/1 -> Rate Transition/1
  Sum/1 -> PID Controller/1
  Rate Transition/1 -> iq_ref/1, [iq_ref]
  w_ref/1 -> Sum/1
  w_meas/1 -> Sum/2

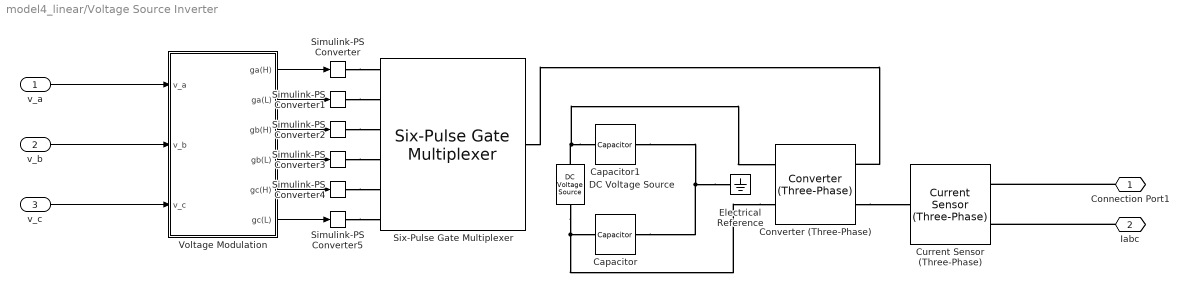
== system model4_linear/Voltage Source Inverter ==
  v_a : Inport
  v_b : Inport  Port=2
  v_c : Inport  Port=3
  Capacitor : ee_lib/Passive/Capacitor  cap_option=ee.enum.passive.capacitor.capOption.const  c=1e-3 F  Cvec=[1e-05, 1e-06] F  Vvec=[0, 10] V  CV_table_symmetry=ee.enum.passive.capacitor.tableSymmetry.yes  f_vec=[1, 10] kHz  DFext_vec=[.8, 1.2]  enable_C_tol=ee.enum.toleranceApplication.none  averaging_period=0 s  C_tol=5  tol_distribution=ee.enum.toleranceDistribution.uniform  nSigma=4  r=0 Ohm  g=0 1/Ohm  enable_operating_limits=ee.enum.enable.no  operating_limit_action=ee.enum.passive.reportOpLim.warn  max_working_voltage_range=[-25, 25] V  power_rating=1 W  maxTemperature=85 degC  thermalEnable=false  thermalMass=1 J/K  i_specify=off  i_priority=None  i=0 A  i_nominal_specify=off  i_nominal_value=1  i_nominal_unit=A  v_specify=off  v_priority=None  v=0 V  v_nominal_specify=off  v_nominal_value=1  v_nominal_unit=V  vc_specify=on  vc_priority=None  vc=0 V  vc_nominal_specify=off  vc_nominal_value=1  vc_nominal_unit=V  T_specify=off  T_priority=None  T=298.15 K  T_nominal_specify=off  T_nominal_value=1  T_nominal_unit=K
  Capacitor1 : ee_lib/Passive/Capacitor  cap_option=ee.enum.passive.capacitor.capOption.const  c=1e-3 F  Cvec=[1e-05, 1e-06] F  Vvec=[0, 10] V  CV_table_symmetry=ee.enum.passive.capacitor.tableSymmetry.yes  f_vec=[1, 10] kHz  DFext_vec=[.8, 1.2]  enable_C_tol=ee.enum.toleranceApplication.none  averaging_period=0 s  C_tol=5  tol_distribution=ee.enum.toleranceDistribution.uniform  nSigma=4  r=0 Ohm  g=0 1/Ohm  enable_operating_limits=ee.enum.enable.no  operating_limit_action=ee.enum.passive.reportOpLim.warn  max_working_voltage_range=[-25, 25] V  power_rating=1 W  maxTemperature=85 degC  thermalEnable=false  thermalMass=1 J/K  i_specify=off  i_priority=None  i=0 A  i_nominal_specify=off  i_nominal_value=1  i_nominal_unit=A  v_specify=off  v_priority=None  v=0 V  v_nominal_specify=off  v_nominal_value=1  v_nominal_unit=V  vc_specify=on  vc_priority=None  vc=0 V  vc_nominal_specify=off  vc_nominal_value=1  vc_nominal_unit=V  T_specify=off  T_priority=None  T=298.15 K  T_nominal_specify=off  T_nominal_value=1  T_nominal_unit=K
  Converter (Three-Phase) : ee_lib/Semiconductors & Converters/Converters/Converter (Three-Phase)  port_option=ee.enum.threePhasePort.composite  fidelity_option=ee.enum.converters.fidelity.detailed  device_type=ee.enum.converters.switchingdevice.averaged  showThermalPort=false  K=0  Vth=6 V  Vgt=1 V  Vgt_off=-1 V  Ih=1 A  Vf=0.8 V  Ron=0.001 Ohm  Rds=0.001 Ohm  Goff=1e-6 1/Ohm  Eon_scalar=22.86e-3 J  Eoff_scalar=17.14e-3 J  Eoff_natural_commutation=10e-3 J  Voff=300 V  Iout_scalar=600 A  onCurrentMeasDelay=0 s  useCurrentFromPreviousCycle=false  useVoltageFromPreviousCycle=false  diode_param=ee.enum.converters.protectiondiode.none  diode_Vf=0.8 V  diode_Ron=0.001 Ohm  diode_Goff=1e-5 1/Ohm  diode_C=50 nF  diode_iRM=-235 A  diode_iF=300 A  diode_idot=-50 A/us  diode_trr_param=ee.enum.converters.diodetrr.trr_factor  diode_trr_factor=3  diode_trr=15 us  diode_Qrr=1500 s*uA  diode_rec_loss_model=ee.enum.diode.reverseRecoveryModel.fixed  diode_ErecVal=0 J  diode_scaleWithIandV=false  diode_ErecMat=zeros(2, 3) J  diode_TjrecVec=[298.15, 398.15] K  diode_IfrecVec=[.1, 1, 10] A  diode_IrecVal=10 A  diode_VrecVal=10 V  diode_tFilter=1 / 1000 / 100 s  thermal_network_parameterization=ee.enum.thermalNetworkTopology.external  Rth=[.08, .5] K/W  Rth_Cauer=[.08, .1, .5] K/W  Rth_Foster=[.08, .14, .22, .16] K/W  thermal_mass_parameterization=ee.enum.thermalNetwork.timeconstant  thermal_mass=[.01, .5] J/K  thermal_mass_Cauer=[.01, .1, .5] J/K  thermal_mass_Foster=[.001, .005, .05, .5] J/K  thermal_time_constant=[.001, .2] s  thermal_time_constant_Cauer=[.001, .1, .2] s  thermal_time_constant_Foster=[7e-05, .0007, .01, .08] s  thermal_mass_initial_temperatures=[25, 25] degC  thermal_mass_initial_temperatures_Cauer=[25, 25, 25] degC  junction_thermal_mass=0.01 J/K  Tvec_initial_Foster=[25, 25, 25, 25] degC  snubber_type=ee.enum.converters.snubber.exclude  Cs=1e-7 F  Rs=0.1 Ohm  Vce_loss=[0, 150, 300] V
  Current Sensor (Three-Phase) : ee_lib/Sensors & Transducers/Current Sensor (Three-Phase)
  DC Voltage Source : ee_lib/Additional Components/SPICE Sources/DC Voltage Source  DC=lin_dc_voltage_source V
  Electrical Reference : fl_lib/Electrical/Electrical Elements/Electrical Reference
  Simulink-PS Converter{,1..5} (6 alike) : nesl_utility/Simulink-PS Converter  PhysicalDomain=network_engine_domain  SubClassName=ps_input  LeftPortType=input  RightPortType=output  PseudoPeriodic=off  Frequencies=[]  NoiseDistribution=none  NoiseParameters=[]  Unit=1  AffineConversion=off  FilteringAndDerivatives=provide  SimscapeFilterOrder=1  InputFilterTimeConstant=0.001  UdotUserProvided=0
  Six-Pulse Gate Multiplexer : ee_lib/Semiconductors & Converters/Converters/Six-Pulse Gate Multiplexer  port_option=ee.enum.controlport.ps
  Voltage Modulation : Subsystem
  Connection Port1 : PMIOPort  Side=Right
  Iabc : PMIOPort  Port=2  Side=Right
  wires:
  Voltage Modulation/1(ga(H)) -> Simulink-PS Converter/1
  Voltage Modulation/6(gc(L)) -> Simulink-PS Converter5/1
  Voltage Modulation/4(gb(L)) -> Simulink-PS Converter3/1
  v_a/1 -> Voltage Modulation/1(v_a)
  Voltage Modulation/3(gb(H)) -> Simulink-PS Converter2/1
  Voltage Modulation/5(gc(H)) -> Simulink-PS Converter4/1
  v_b/1 -> Voltage Modulation/2(v_b)
  v_c/1 -> Voltage Modulation/3(v_c)
  Voltage Modulation/2(ga(L)) -> Simulink-PS Converter1/1
  connections:
  Electrical Reference/LConn1 -- Capacitor1/RConn1 -- Capacitor/LConn1
  Capacitor1/LConn1 -- DC Voltage Source/LConn1 -- Converter (Three-Phase)/RConn1
  Converter (Three-Phase)/RConn2 -- DC Voltage Source/RConn1 -- Capacitor/RConn1
  Simulink-PS Converter4/RConn1 -- Six-Pulse Gate Multiplexer/LConn5
  Converter (Three-Phase)/LConn2 -- Current Sensor (Three-Phase)/LConn1
  Simulink-PS Converter/RConn1 -- Six-Pulse Gate Multiplexer/LConn1
  Simulink-PS Converter1/RConn1 -- Six-Pulse Gate Multiplexer/LConn2
  Iabc/RConn1 -- Current Sensor (Three-Phase)/RConn1
  Connection Port1/RConn1 -- Current Sensor (Three-Phase)/RConn2
  Simulink-PS Converter2/RConn1 -- Six-Pulse Gate Multiplexer/LConn3
  Six-Pulse Gate Multiplexer/RConn1 -- Converter (Three-Phase)/LConn1
  Simulink-PS Converter5/RConn1 -- Six-Pulse Gate Multiplexer/LConn6
  Simulink-PS Converter3/RConn1 -- Six-Pulse Gate Multiplexer/LConn4

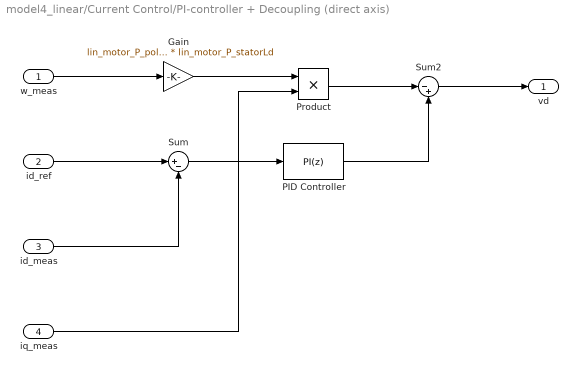
== system model4_linear/Current Control/PI-controller + Decoupling (direct axis) ==
  w_meas : Inport
  id_ref : Inport  Port=2
  id_meas : Inport  Port=3
  iq_meas : Inport  Port=4
  Gain : Gain  Gain=lin_motor_P_pole_pairs * lin_motor_P_statorLd
  PID Controller : slpidlib/PID Controller  Controller=PI  Form=Parallel  TimeDomain=Discrete-time  UseExternalTs=off  SampleTime=current_con_ts  IntegratorMethod=Forward Euler  FilterMethod=Forward Euler  ControllerParametersSource=internal  P=lin_current_con_Kp  I=lin_current_con_Ki  UseKiTs=off  D=0  UseExternalDerivativeSource=off  N=100  UseFilter=on  TunerSelectOption=Transfer Function Based (PID Tuner App)  InitialConditionSource=internal  InitialConditionForIntegrator=0  InitialConditionForFilter=0  DifferentiatorICPrevScaledInput=0  ExternalReset=none  TrackingMode=off  Kt=1  LimitOutput=on  SatLimitsSource=internal  UpperSaturationLimit=18  LowerSaturationLimit=-18  LinearizeAsGain=on  AntiWindupMode=clamping  Kb=1  LimitIntegrator=off  UpperIntegratorSaturationLimit=inf  LowerIntegratorSaturationLimit=-inf  POutMin=[]  POutMax=[]  IOutMin=[]  IOutMax=[]  DOutMin=[]  DOutMax=[]  NOutMin=[]  NOutMax=[]  SumOutMin=[]  SumOutMax=[]  SaturationOutMin=[]  SaturationOutMax=[]  PParamMin=[]  PParamMax=[]  IParamMin=[]  IParamMax=[]  DParamMin=[]  DParamMax=[]  NParamMin=[]  NParamMax=[]  KbParamMin=[]  KbParamMax=[]  KtParamMin=[]  KtParamMax=[]  KbOutMin=[]  KbOutMax=[]  KtOutMin=[]  KtOutMax=[]  IntegratorOutMin=[]  IntegratorOutMax=[]  FilterOutMin=[]  FilterOutMax=[]  SumI1OutMin=[]  SumI1OutMax=[]  SumI2OutMin=[]  SumI2OutMax=[]  SumI3OutMin=[]  SumI3OutMax=[]  SumI4OutMin=[]  SumI4OutMax=[]  SumDOutMin=[]  SumDOutMax=[]  DifferentiatorOutMin=[]  DifferentiatorOutMax=[]  FilterDiffOutCoefMin=[]  FilterDiffOutCoefMax=[]  ReciprocalOutMin=[]  ReciprocalOutMax=[]  SumDenOutMin=[]  SumDenOutMax=[]  SumNumOutMin=[]  SumNumOutMax=[]  DivideOutMin=[]  DivideOutMax=[]  UdiffTsProdOutMin=[]  UdiffTsProdOutMax=[]  NTsProdOutMin=[]  NTsProdOutMax=[]  UintegralTsProdOutMin=[]  UintegralTsProdOutMax=[]  UngainTsProdOutMin=[]  UngainTsProdOutMax=[]  ClampingZeroOutDataTypeStr=Inherit: Inherit via back propagation  ClampingZeroOutMin=[]  ClampingZeroOutMax=[]  FilterDenConstantOutDataTypeStr=Inherit: Inherit via back propagation  FilterDenConstantOutMin=[]  FilterDenConstantOutMax=[]  PCopyOutDataTypeStr=Inherit: Inherit via back propagation  PCopyOutMin=[]  PCopyOutMax=[]  NCopyOutDataTypeStr=Inherit: Inherit via back propagation  NCopyOutMin=[]  NCopyOutMax=[]  IntegratorContinuousStateAttributes=''  IntegratorStateMustResolveToSignalObject=off  IntegratorRTWStateStorageClass=Auto  FilterContinuousStateAttributes=''  FilterStateMustResolveToSignalObject=off  FilterRTWStateStorageClass=Auto  ParallelPVariant=InternalParameters  IdealPVariant=Disabled  IVariant=InternalParameters  DVariant=Disabled  IntegratorVariant=Discrete  SatVariant=Enabled  AWVariant=DiscClampingParallel  PCopyVariant=Disabled  TRVariant=Disabled  FdbkBlocksVariant=Forward  IdealPFdbkVariant=Disabled  SatFdbkVariant=Disabled  DerivativeFilterVariant=Disabled  NVariant=Disabled  NCopyVariant=Disabled_SignalSpec  FilterICVariant=Disabled  IntegratorICVariant=InternalICs  ExternalResetVariant=Disabled  TRSumVariant=Passthrough  SumFdbkVariant=Disabled  SumVariant=Sum_PI  TsampFilterVariant=InternalTs  TsampNgainVariant=Passthrough  TsampIntegralVariant=Disabled_SignalSpec  ExternalSaturationOutDataTypeStr=Inherit: Same as second input  DerivativeSourceVariant=Disabled  PreIntVariant=InternalPreInt
  Product : Product
  Sum : Sum  Inputs=|+-
  Sum2 : Sum  Inputs=|-+
  vd : Outport
  wires:
  PID Controller/1 -> Sum2/2
  w_meas/1 -> Gain/1
  id_ref/1 -> Sum/1
  id_meas/1 -> Sum/2
  Gain/1 -> Product/1
  Sum/1 -> PID Controller/1
  Product/1 -> Sum2/1
  iq_meas/1 -> Product/2
  Sum2/1 -> vd/1

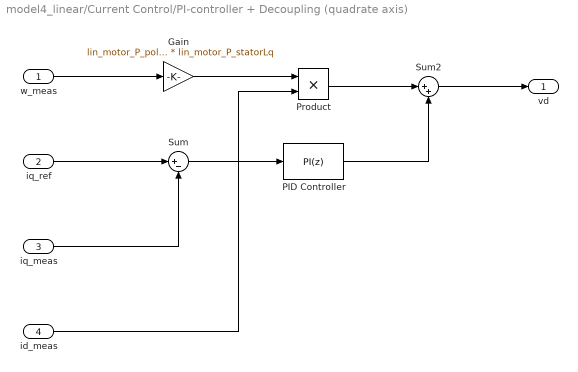
== system model4_linear/Current Control/PI-controller + Decoupling (quadrate axis) ==
  w_meas : Inport
  iq_ref : Inport  Port=2
  iq_meas : Inport  Port=3
  id_meas : Inport  Port=4
  Gain : Gain  Gain=lin_motor_P_pole_pairs * lin_motor_P_statorLq
  PID Controller : slpidlib/PID Controller  Controller=PI  Form=Parallel  TimeDomain=Discrete-time  UseExternalTs=off  SampleTime=current_con_ts  IntegratorMethod=Forward Euler  FilterMethod=Forward Euler  ControllerParametersSource=internal  P=lin_current_con_Kp  I=lin_current_con_Ki  UseKiTs=off  D=0  UseExternalDerivativeSource=off  N=100  UseFilter=on  TunerSelectOption=Transfer Function Based (PID Tuner App)  InitialConditionSource=internal  InitialConditionForIntegrator=0  InitialConditionForFilter=0  DifferentiatorICPrevScaledInput=0  ExternalReset=none  TrackingMode=off  Kt=1  LimitOutput=on  SatLimitsSource=internal  UpperSaturationLimit=18  LowerSaturationLimit=-18  LinearizeAsGain=on  AntiWindupMode=clamping  Kb=1  LimitIntegrator=off  UpperIntegratorSaturationLimit=inf  LowerIntegratorSaturationLimit=-inf  POutMin=[]  POutMax=[]  IOutMin=[]  IOutMax=[]  DOutMin=[]  DOutMax=[]  NOutMin=[]  NOutMax=[]  SumOutMin=[]  SumOutMax=[]  SaturationOutMin=[]  SaturationOutMax=[]  PParamMin=[]  PParamMax=[]  IParamMin=[]  IParamMax=[]  DParamMin=[]  DParamMax=[]  NParamMin=[]  NParamMax=[]  KbParamMin=[]  KbParamMax=[]  KtParamMin=[]  KtParamMax=[]  KbOutMin=[]  KbOutMax=[]  KtOutMin=[]  KtOutMax=[]  IntegratorOutMin=[]  IntegratorOutMax=[]  FilterOutMin=[]  FilterOutMax=[]  SumI1OutMin=[]  SumI1OutMax=[]  SumI2OutMin=[]  SumI2OutMax=[]  SumI3OutMin=[]  SumI3OutMax=[]  SumI4OutMin=[]  SumI4OutMax=[]  SumDOutMin=[]  SumDOutMax=[]  DifferentiatorOutMin=[]  DifferentiatorOutMax=[]  FilterDiffOutCoefMin=[]  FilterDiffOutCoefMax=[]  ReciprocalOutMin=[]  ReciprocalOutMax=[]  SumDenOutMin=[]  SumDenOutMax=[]  SumNumOutMin=[]  SumNumOutMax=[]  DivideOutMin=[]  DivideOutMax=[]  UdiffTsProdOutMin=[]  UdiffTsProdOutMax=[]  NTsProdOutMin=[]  NTsProdOutMax=[]  UintegralTsProdOutMin=[]  UintegralTsProdOutMax=[]  UngainTsProdOutMin=[]  UngainTsProdOutMax=[]  ClampingZeroOutDataTypeStr=Inherit: Inherit via back propagation  ClampingZeroOutMin=[]  ClampingZeroOutMax=[]  FilterDenConstantOutDataTypeStr=Inherit: Inherit via back propagation  FilterDenConstantOutMin=[]  FilterDenConstantOutMax=[]  PCopyOutDataTypeStr=Inherit: Inherit via back propagation  PCopyOutMin=[]  PCopyOutMax=[]  NCopyOutDataTypeStr=Inherit: Inherit via back propagation  NCopyOutMin=[]  NCopyOutMax=[]  IntegratorContinuousStateAttributes=''  IntegratorStateMustResolveToSignalObject=off  IntegratorRTWStateStorageClass=Auto  FilterContinuousStateAttributes=''  FilterStateMustResolveToSignalObject=off  FilterRTWStateStorageClass=Auto  ParallelPVariant=InternalParameters  IdealPVariant=Disabled  IVariant=InternalParameters  DVariant=Disabled  IntegratorVariant=Discrete  SatVariant=Enabled  AWVariant=DiscClampingParallel  PCopyVariant=Disabled  TRVariant=Disabled  FdbkBlocksVariant=Forward  IdealPFdbkVariant=Disabled  SatFdbkVariant=Disabled  DerivativeFilterVariant=Disabled  NVariant=Disabled  NCopyVariant=Disabled_SignalSpec  FilterICVariant=Disabled  IntegratorICVariant=InternalICs  ExternalResetVariant=Disabled  TRSumVariant=Passthrough  SumFdbkVariant=Disabled  SumVariant=Sum_PI  TsampFilterVariant=InternalTs  TsampNgainVariant=Passthrough  TsampIntegralVariant=Disabled_SignalSpec  ExternalSaturationOutDataTypeStr=Inherit: Same as second input  DerivativeSourceVariant=Disabled  PreIntVariant=InternalPreInt
  Product : Product
  Sum : Sum  Inputs=|+-
  Sum2 : Sum  Inputs=|++
  vd : Outport
  wires:
  PID Controller/1 -> Sum2/2
  w_meas/1 -> Gain/1
  iq_ref/1 -> Sum/1
  iq_meas/1 -> Sum/2
  Gain/1 -> Product/1
  Sum/1 -> PID Controller/1
  Product/1 -> Sum2/1
  id_meas/1 -> Product/2
  Sum2/1 -> vd/1

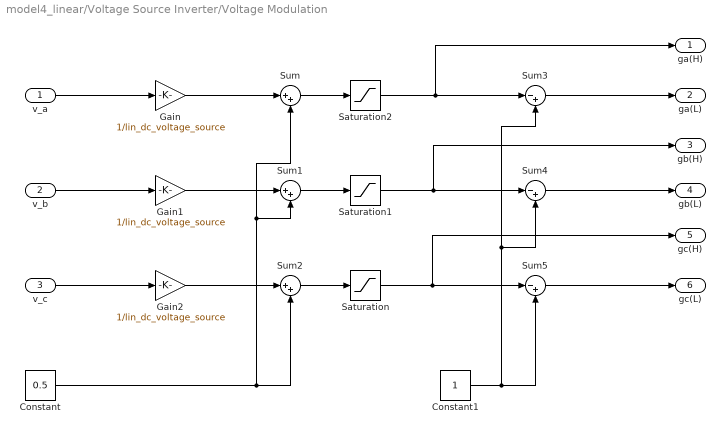
== system model4_linear/Voltage Source Inverter/Voltage Modulation ==
  v_a : Inport
  v_b : Inport  Port=2
  v_c : Inport  Port=3
  Constant : Constant  Value=0.5
  Constant1 : Constant
  Gain : Gain  Gain=1/lin_dc_voltage_source
  Gain1 : Gain  Gain=1/lin_dc_voltage_source
  Gain2 : Gain  Gain=1/lin_dc_voltage_source
  Saturation : Saturate  UpperLimit=1  LowerLimit=0
  Saturation1 : Saturate  UpperLimit=1  LowerLimit=0
  Saturation2 : Saturate  UpperLimit=1  LowerLimit=0
  Sum : Sum  Inputs=|++
  Sum1 : Sum  Inputs=|++
  Sum2 : Sum  Inputs=|++
  Sum3 : Sum  Inputs=|-+
  Sum4 : Sum  Inputs=|-+
  Sum5 : Sum  Inputs=|-+
  ga(H) : Outport
  ga(L) : Outport  Port=2
  gb(H) : Outport  Port=3
  gb(L) : Outport  Port=4
  gc(H) : Outport  Port=5
  gc(L) : Outport  Port=6
  wires:
  v_a/1 -> Gain/1
  v_b/1 -> Gain1/1
  v_c/1 -> Gain2/1
  Constant/1 -> Sum/2, Sum1/2, Sum2/2
  Gain/1 -> Sum/1
  Gain1/1 -> Sum1/1
  Gain2/1 -> Sum2/1
  Sum2/1 -> Saturation/1
  Sum1/1 -> Saturation1/1
  Sum/1 -> Saturation2/1
  Constant1/1 -> Sum5/2, Sum3/2, Sum4/2
  Sum3/1 -> ga(L)/1
  Sum4/1 -> gb(L)/1
  Sum5/1 -> gc(L)/1
  Saturation/1 -> gc(H)/1, Sum5/1
  Saturation1/1 -> gb(H)/1, Sum4/1
  Saturation2/1 -> ga(H)/1, Sum3/1
